simulink model "SpeedToPulse"  (R2014a)
settings: Solver=FixedStepDiscrete  StartTime=0.0  StopTime=100000  FixedStep=1  RelTol=1e-3
libraries: hdlsllib x1
settings Model: Creator=rogers.a  LastModifiedBy=rogers.a

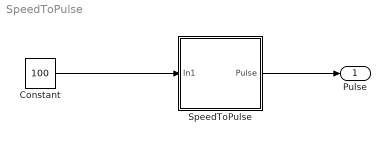
== system SpeedToPulse ==
  Constant : Constant  Value=100  OutDataTypeStr=int8
  SpeedToPulse : Subsystem
  Pulse : Outport
  wires:
  Constant/1 -> SpeedToPulse/1(In1)
  SpeedToPulse/1(Pulse) -> Pulse/1

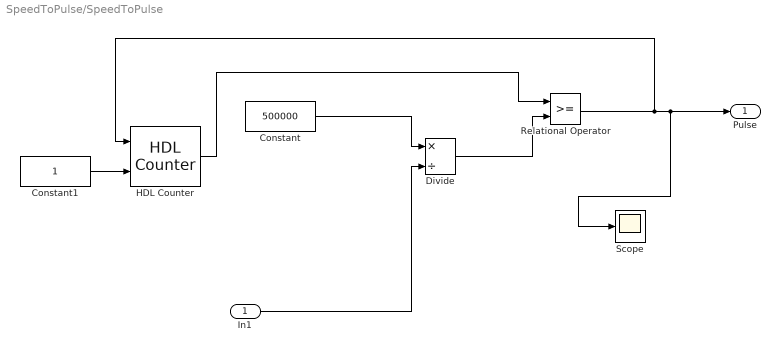
== system SpeedToPulse/SpeedToPulse ==
  In1 : Inport
  Constant : Constant  Value=500000  OutDataTypeStr=int32
  Constant1 : Constant  OutDataTypeStr=boolean
  Divide : Product  Inputs=*/  SaturateOnIntegerOverflow=on  RndMeth=Zero
  HDL Counter : hdlsllib/HDL Operations/HDL Counter  CountType=Free running  CountInit=0  CountStep=1  CountMax=10000  CountFromType=Initial value  CountFrom=0  CountResetPort=on  CountLoadPort=off  CountEnbPort=on  CountDirPort=off  CountDataType=Unsigned  CountWordLen=32  CountFracLen=0  CountSampTime=1
  Relational Operator : RelationalOperator  OutDataTypeStr=boolean
  Scope : Scope
  Pulse : Outport
  wires:
  HDL Counter/1 -> Relational Operator/1
  Constant/1 -> Divide/1
  Divide/1 -> Relational Operator/2
  In1/1 -> Divide/2
  Relational Operator/1 -> Pulse/1, Scope/1, HDL Counter/1
  Constant1/1 -> HDL Counter/2
